simulink subsystem "error_flag_generator"  (R2019b)
settings: Solver=VariableStepAuto  StartTime=0.0  StopTime=10.0  RelTol=1e-3
settings Model: Creator=andrea  LastModifiedBy=matildeiuculano

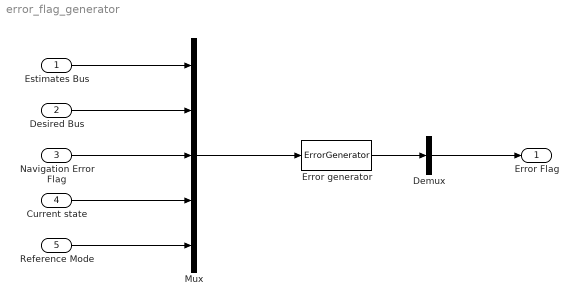
== system error_flag_generator ==
  Estimates Bus : Inport
  Desired Bus : Inport  Port=2
  Navigation Error Flag : Inport  Port=3
  "Current state " : Inport  Port=4
  "Reference Mode " : Inport  Port=5
  Demux : Demux  Outputs=1
  Error generator : MATLABFcn  MATLABFcn=ErrorGenerator
  Mux : Mux  Inputs=5
  Error Flag : Outport
  wires:
  Demux/1 -> Error Flag/1
  Error generator/1 -> Demux/1
  "Current state "/1 -> Mux/4
  Navigation Error Flag/1 -> Mux/3
  Mux/1 -> Error generator/1
  "Reference Mode "/1 -> Mux/5
  Desired Bus/1 -> Mux/2
  Estimates Bus/1 -> Mux/1
